simulink model "vehicle_lat_dyn_sim"  (Simulink 9.1)
settings: Solver=ode45  StartTime=0.0  StopTime=Tend  RelTol=1e-3
values from neighbouring files (symbols this model uses):
  alfaf0 = 0    [dati2.m]    (also in vehicle_lat_dyn_main.m)
  alfar0 = 0    [dati2.m]    (also in vehicle_lat_dyn_main.m)
  bf = 12    [data_vehicle.m]    (also in dati.m; dati2.m)
  br = 14    [data_vehicle.m]    (also in dati.m = 18; dati2.m = 18)
  Cd = .3    (= 0.3)    [data_vehicle.m]    (also in dati.m; dati2.m)
  Cf = 1.3    [data_vehicle.m]    (also in dati.m; dati2.m)
  Cr = 1.3    [data_vehicle.m]    (also in dati.m; dati2.m)
  df = 0.95    [data_vehicle.m]    (also in dati.m; dati2.m)
  dr = 1    [data_vehicle.m]    (also in dati.m = 1.1; dati2.m = 1.1)
  dt_save = 1e-2    (= 0.01)    [dati2.m]    (also in vehicle_lat_dyn_main.m)
  Ef = -0.1    [data_vehicle.m]    (also in dati.m; dati2.m)
  Er = -0.1    [data_vehicle.m]    (also in dati.m; dati2.m)
  fv = .02    (= 0.02)    [data_vehicle.m]    (also in dati.m; dati2.m)
  Fzf = m*g*lr/l    [data_vehicle.m]    (also in dati.m = 9879.29185185; dati2.m = 9879.29185185)
  Fzr = m*g*lf/l    [data_vehicle.m]    (also in dati.m = 5811.34814815; dati2.m = 5811.34814815)
  g = 9.80665    [dati.m]    (also in dati2.m; vehicle_lat_dyn_main.m)
  gB = 2/3    (= 0.666666666667)    [data_vehicle.m]    (also in dati.m; dati2.m)
  gT = 0    [data_vehicle.m]    (also in dati.m = 1; dati2.m = 1)
  Jz = 2200    [data_vehicle.m]    (also in dati.m; dati2.m)
  L = 2    [data_vehicle.m]    (also in dati.m; dati2.m)
  lf = 1    [data_vehicle.m]    (also in dati.m; dati2.m)
  lr = l-lf    (= 1.7)    [data_vehicle.m]    (also in dati.m; dati2.m)
  m = 1600    [data_vehicle.m]    (also in dati.m; dati2.m)
  mu = 1    [data_vehicle.m]    (also in dati.m; dati2.m)
  psi0 = 0    [dati2.m]    (also in vehicle_lat_dyn_main.m)
  psip0 = 0    [dati2.m]    (also in vehicle_lat_dyn_main.m)
  rho = 1.2    [data_vehicle.m]    (also in dati.m; dati2.m)
  S = 2    [data_vehicle.m]    (also in dati.m; dati2.m)
  vy0 = 0    [dati2.m]    (also in vehicle_lat_dyn_main.m)
  XG0 = 0    [dati2.m]    (also in vehicle_lat_dyn_main.m)
  YG0 = 0    [dati2.m]    (also in vehicle_lat_dyn_main.m)
undefined symbols (not defined in the file or in its folder): axh, deltah, vxh
settings Model: Creator=mic  LastModifiedBy=jdrjk
settings DataIOCC: SaveFormat=StructureWithTime  SaveOutput=off  SignalLogging=off  DSMLogging=off  OutputOption=SpecifiedOutputTimes  OutputTimes=[0:dt_save:Tend]
settings DebuggingCC: UnderspecifiedInitializationDetection=Simplified  MergeDetectMultiDrivingBlocksExec=error  SFUnexpectedBacktrackingDiag=error  SFNoUnconditionalDefaultTransitionDiag=error
settings HardwareCC: ProdBitPerPointer=64  ProdLargestAtomicFloat=Float  ProdIntDivRoundTo=Zero  ProdEndianess=LittleEndian  ProdHWDeviceType=Specified
settings ModelReferenceCC: PropagateSignalLabelsOutOfModel=on
settings GRTTargetCC: TargetLangStandard=C99 (ISO)  CombineOutputUpdateFcns=on  GRTInterface=off
settings ConfigComp: CovMetricSettings=dwe  CovHtmlReporting=off  CovSaveCumulativeToWorkspaceVar=off  CovSaveSingleToWorkspaceVar=off  CovExternalEMLEnable=on

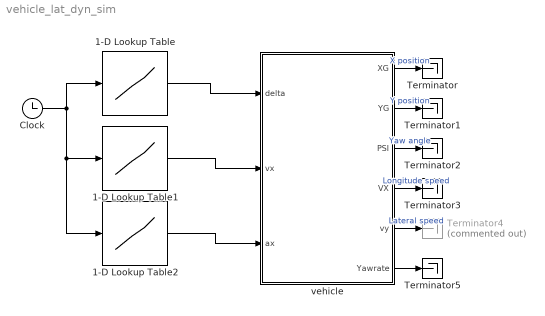
== system vehicle_lat_dyn_sim ==
  1-D Lookup Table : Lookup_n-D  NumberOfTableDimensions=1  BreakpointsForDimension1=deltah(:,1)  Table=deltah(:,2)  RndMeth=Simplest  InputSameDT=on
  1-D Lookup Table1 : Lookup_n-D  NumberOfTableDimensions=1  BreakpointsForDimension1=vxh(:,1)  Table=vxh(:,2)  RndMeth=Simplest  InputSameDT=on
  1-D Lookup Table2 : Lookup_n-D  NumberOfTableDimensions=1  BreakpointsForDimension1=axh(:,1)  Table=axh(:,2)  RndMeth=Simplest  InputSameDT=on
  Clock : Clock
  Terminator{,1..3,5} (5 alike) : Terminator
  Terminator4 : Terminator  Commented=on
  vehicle : Subsystem
  wires:
  Clock/1 -> 1-D Lookup Table2/1, 1-D Lookup Table1/1, 1-D Lookup Table/1
  1-D Lookup Table1/1 -> vehicle/2(vx)
  1-D Lookup Table2/1 -> vehicle/3(ax)
  1-D Lookup Table/1 -> vehicle/1(delta)
  vehicle/1(XG) -> Terminator/1  "X position"
  vehicle/2(YG) -> Terminator1/1  "Y position"
  vehicle/3(PSI) -> Terminator2/1  "Yaw angle"
  vehicle/4(VX) -> Terminator3/1  "Longitude speed"
  vehicle/5(vy) -> Terminator4/1  "Lateral speed"
  vehicle/6("Yawrate ") -> Terminator5/1

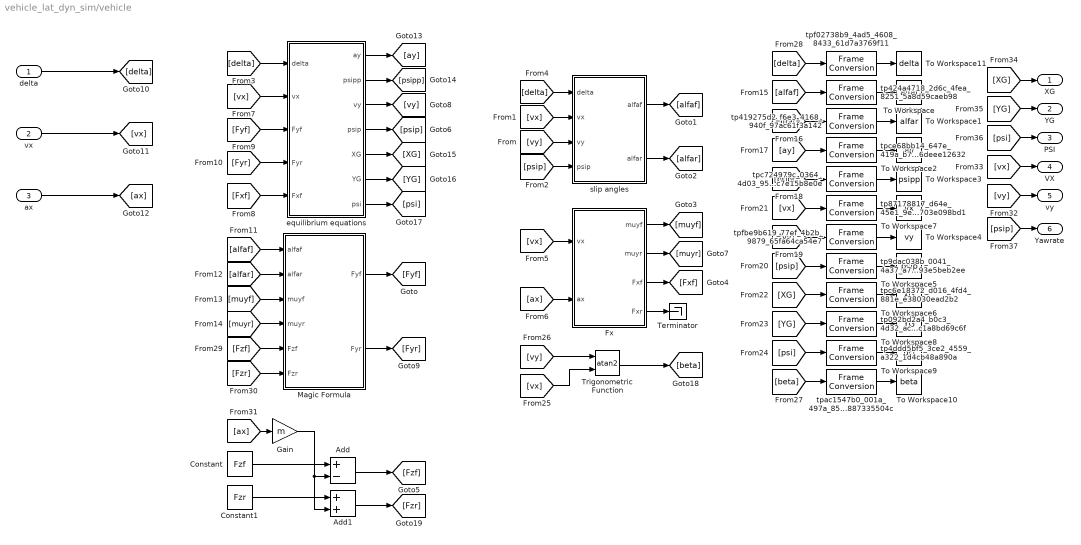
== system vehicle_lat_dyn_sim/vehicle ==
  delta : Inport
  vx : Inport  Port=2
  ax : Inport  Port=3
  Add : Sum  Inputs=+-
  Add1 : Sum
  Constant : Constant  Value=Fzf
  Constant1 : Constant  Value=Fzr
  Fx : Subsystem
  Gain : Gain  Gain=m
  Magic Formula : Subsystem
  Terminator : Terminator
  To Workspace : ToWorkspace  VariableName=alfaf  SampleTime=dt_save
  To Workspace1 : ToWorkspace  VariableName=alfar  SampleTime=dt_save
  To Workspace10 : ToWorkspace  VariableName=beta  SampleTime=dt_save
  To Workspace11 : ToWorkspace  VariableName=delta  SampleTime=dt_save
  To Workspace2 : ToWorkspace  VariableName=ay  SampleTime=dt_save
  To Workspace3 : ToWorkspace  VariableName=psipp  SampleTime=dt_save
  To Workspace4 : ToWorkspace  VariableName=vy  SampleTime=dt_save
  To Workspace5 : ToWorkspace  VariableName=psip  SampleTime=dt_save
  To Workspace6 : ToWorkspace  VariableName=XG  SampleTime=dt_save
  To Workspace7 : ToWorkspace  VariableName=vx  SampleTime=dt_save
  To Workspace8 : ToWorkspace  VariableName=YG  SampleTime=dt_save
  To Workspace9 : ToWorkspace  VariableName=psi  SampleTime=dt_save
  Trigonometric Function : Trigonometry  Operator=atan2
  equilibrium equations : Subsystem
  slip angles : Subsystem
  tp092bd2a4_b0c3_4d32_ac59_7c1a8bd69c6f : FrameConversion  OutFrame=Sample-based
  tp419275d2_f6e3_4168_940f_97ac61f3a142 : FrameConversion  OutFrame=Sample-based
  tp424a4718_2d6c_4fea_8251_5a8d59caeb98 : FrameConversion  OutFrame=Sample-based
  tp4ddd5bf5_3ce2_4559_a322_1d4cb48a890a : FrameConversion  OutFrame=Sample-based
  tp87178817_d64e_45e1_9e30_db703e098bd1 : FrameConversion  OutFrame=Sample-based
  tp9dac038b_0041_4a37_a752_0593e5beb2ee : FrameConversion  OutFrame=Sample-based
  tpac1547b0_001a_497a_857c_68887335504c : FrameConversion  OutFrame=Sample-based
  tpc6e18372_d016_4fd4_881e_e38030ead2b2 : FrameConversion  OutFrame=Sample-based
  tpc724979c_0364_4d03_952a_37c7e15b8e0e : FrameConversion  OutFrame=Sample-based
  tpce68bb14_647e_419a_b744_5f6deee12632 : FrameConversion  OutFrame=Sample-based
  tpf02738b9_4ad5_4608_8433_61d7a3769f11 : FrameConversion  OutFrame=Sample-based
  tpfbe9b619_77ef_4b2b_9879_65fa64ca54e7 : FrameConversion  OutFrame=Sample-based
  XG : Outport
  YG : Outport  Port=2
  PSI : Outport  Port=3
  VX : Outport  Port=4
  vy : Outport  Port=5
  "Yawrate " : Outport  Port=6
  wires:
  [vx] -> VX/1
  [psi] -> PSI/1
  [XG] -> XG/1
  [YG] -> YG/1
  [vy] -> vy/1
  [vx] -> equilibrium equations/2(vx)
  Magic Formula/2(Fyr) -> [Fyr]
  slip angles/1(alfaf) -> [alfaf]
  equilibrium equations/4(psip) -> [psip]
  [delta] -> equilibrium equations/1(delta)
  [vx] -> slip angles/2(vx)
  [ax] -> Fx/2(ax)
  Fx/4(Fxr) -> Terminator/1
  [Fxf] -> equilibrium equations/5(Fxf)
  [alfar] -> Magic Formula/2(alfar)
  [muyf] -> Magic Formula/3(muyf)
  [vy] -> slip angles/3(vy)
  [muyr] -> Magic Formula/4(muyr)
  slip angles/2(alfar) -> [alfar]
  Magic Formula/1(Fyf) -> [Fyf]
  [Fyf] -> equilibrium equations/3(Fyf)
  equilibrium equations/3(vy) -> [vy]
  [psip] -> slip angles/4(psip)
  [Fyr] -> equilibrium equations/4(Fyr)
  [vx] -> Fx/1(vx)
  delta/1 -> [delta]
  vx/1 -> [vx]
  Fx/1(muyf) -> [muyf]
  [alfaf] -> Magic Formula/1(alfaf)
  [delta] -> slip angles/1(delta)
  Fx/2(muyr) -> [muyr]
  Fx/3(Fxf) -> [Fxf]
  [delta] -> tpf02738b9_4ad5_4608_8433_61d7a3769f11/1
  tpf02738b9_4ad5_4608_8433_61d7a3769f11/1 -> To Workspace11/1
  [ay] -> tpce68bb14_647e_419a_b744_5f6deee12632/1
  equilibrium equations/7(psi) -> [psi]
  ax/1 -> [ax]
  [alfar] -> tp419275d2_f6e3_4168_940f_97ac61f3a142/1
  [alfaf] -> tp424a4718_2d6c_4fea_8251_5a8d59caeb98/1
  tpce68bb14_647e_419a_b744_5f6deee12632/1 -> To Workspace2/1
  [psipp] -> tpc724979c_0364_4d03_952a_37c7e15b8e0e/1
  equilibrium equations/2(psipp) -> [psipp]
  [vy] -> Trigonometric Function/1
  [Fzf] -> Magic Formula/5(Fzf)
  Gain/1 -> Add1/2, Add/2
  tp424a4718_2d6c_4fea_8251_5a8d59caeb98/1 -> To Workspace/1
  [beta] -> tpac1547b0_001a_497a_857c_68887335504c/1
  equilibrium equations/6(YG) -> [YG]
  Add1/1 -> [Fzr]
  tpac1547b0_001a_497a_857c_68887335504c/1 -> To Workspace10/1
  equilibrium equations/1(ay) -> [ay]
  Constant/1 -> Add/1
  equilibrium equations/5(XG) -> [XG]
  Constant1/1 -> Add1/1
  [Fzr] -> Magic Formula/6(Fzr)
  Trigonometric Function/1 -> [beta]
  Add/1 -> [Fzf]
  [vx] -> Trigonometric Function/2
  [ax] -> Gain/1
  tp419275d2_f6e3_4168_940f_97ac61f3a142/1 -> To Workspace1/1
  tp092bd2a4_b0c3_4d32_ac59_7c1a8bd69c6f/1 -> To Workspace8/1
  tp4ddd5bf5_3ce2_4559_a322_1d4cb48a890a/1 -> To Workspace9/1
  tpc724979c_0364_4d03_952a_37c7e15b8e0e/1 -> To Workspace3/1
  [psip] -> tp9dac038b_0041_4a37_a752_0593e5beb2ee/1
  tp87178817_d64e_45e1_9e30_db703e098bd1/1 -> To Workspace7/1
  tpc6e18372_d016_4fd4_881e_e38030ead2b2/1 -> To Workspace6/1
  [vy] -> tpfbe9b619_77ef_4b2b_9879_65fa64ca54e7/1
  tpfbe9b619_77ef_4b2b_9879_65fa64ca54e7/1 -> To Workspace4/1
  [XG] -> tpc6e18372_d016_4fd4_881e_e38030ead2b2/1
  [YG] -> tp092bd2a4_b0c3_4d32_ac59_7c1a8bd69c6f/1
  [vx] -> tp87178817_d64e_45e1_9e30_db703e098bd1/1
  tp9dac038b_0041_4a37_a752_0593e5beb2ee/1 -> To Workspace5/1
  [psi] -> tp4ddd5bf5_3ce2_4559_a322_1d4cb48a890a/1
  [psip] -> "Yawrate "/1

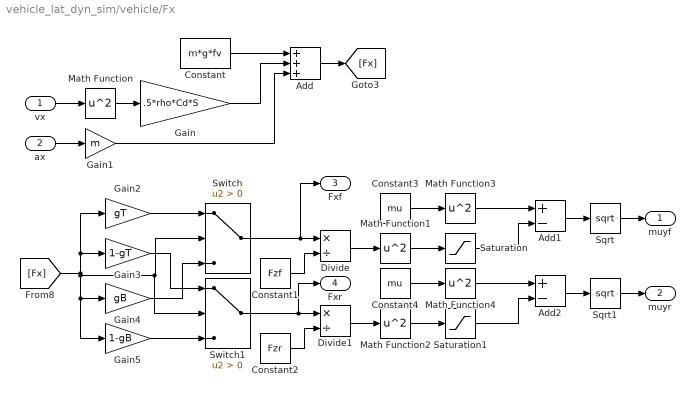
== system vehicle_lat_dyn_sim/vehicle/Fx ==
  vx : Inport
  ax : Inport  Port=2
  Add : Sum  Inputs=+++
  Add1 : Sum  Inputs=+-
  Add2 : Sum  Inputs=+-
  Constant : Constant  Value=m*g*fv
  Constant1 : Constant  Value=Fzf
  Constant2 : Constant  Value=Fzr
  Constant3 : Constant  Value=mu
  Constant4 : Constant  Value=mu
  Divide : Product  Inputs=*/
  Divide1 : Product  Inputs=*/
  Gain : Gain  Gain=.5*rho*Cd*S
  Gain1 : Gain  Gain=m
  Gain2 : Gain  Gain=gT
  Gain3 : Gain  Gain=1-gT
  Gain4 : Gain  Gain=gB
  Gain5 : Gain  Gain=1-gB
  Math Function{,1..4} (5 alike) : Math  Operator=square  SaturateOnIntegerOverflow=on
  Saturation : Saturate  UpperLimit=1  LowerLimit=0
  Saturation1 : Saturate  UpperLimit=1  LowerLimit=0
  Sqrt : Sqrt  SaturateOnIntegerOverflow=on
  Sqrt1 : Sqrt  SaturateOnIntegerOverflow=on
  Switch : Switch  Criteria=u2 > Threshold
  Switch1 : Switch  Criteria=u2 > Threshold
  muyf : Outport
  muyr : Outport  Port=2
  Fxf : Outport  Port=3
  Fxr : Outport  Port=4
  wires:
  Constant/1 -> Add/1
  Gain4/1 -> Switch/3
  Add/1 -> [Fx]
  [Fx] -> Gain2/1, Gain3/1, Switch1/2, Switch/2, Gain5/1, Gain4/1
  Gain3/1 -> Switch1/1
  Gain5/1 -> Switch1/3
  Gain1/1 -> Add/3
  Math Function/1 -> Gain/1
  Gain2/1 -> Switch/1
  Gain/1 -> Add/2
  ax/1 -> Gain1/1
  vx/1 -> Math Function/1
  Switch/1 -> Fxf/1, Divide/1
  Switch1/1 -> Fxr/1, Divide1/1
  Constant1/1 -> Divide/2
  Constant2/1 -> Divide1/2
  Constant3/1 -> Math Function3/1
  Divide/1 -> Math Function1/1
  Divide1/1 -> Math Function2/1
  Math Function1/1 -> Saturation/1
  Math Function2/1 -> Saturation1/1
  Constant4/1 -> Math Function4/1
  Saturation1/1 -> Add2/2
  Saturation/1 -> Add1/2
  Add1/1 -> Sqrt/1
  Add2/1 -> Sqrt1/1
  Sqrt1/1 -> muyr/1
  Sqrt/1 -> muyf/1
  Math Function3/1 -> Add1/1
  Math Function4/1 -> Add2/1

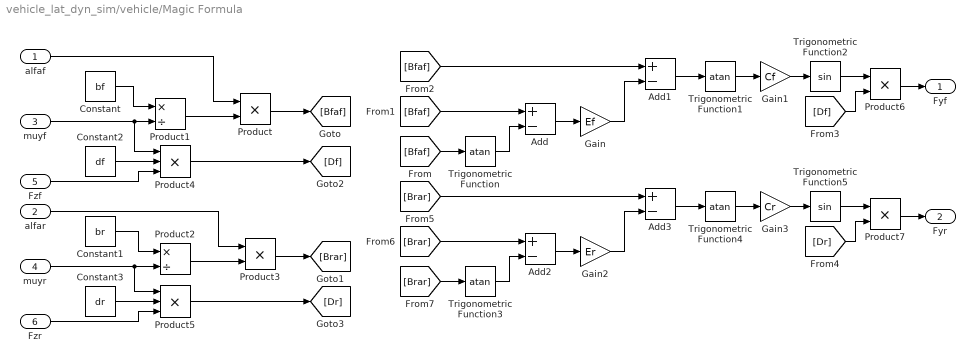
== system vehicle_lat_dyn_sim/vehicle/Magic Formula ==
  alfaf : Inport
  alfar : Inport  Port=2
  muyf : Inport  Port=3
  muyr : Inport  Port=4
  Fzf : Inport  Port=5
  Fzr : Inport  Port=6
  Add{,1..3} (4 alike) : Sum  Inputs=+-
  Constant : Constant  Value=bf
  Constant1 : Constant  Value=br
  Constant2 : Constant  Value=df
  Constant3 : Constant  Value=dr
  Gain : Gain  Gain=Ef
  Gain1 : Gain  Gain=Cf
  Gain2 : Gain  Gain=Er
  Gain3 : Gain  Gain=Cr
  Product{,3,6..7} (4 alike) : Product
  Product1 : Product  Inputs=*/
  Product2 : Product  Inputs=*/
  Product4 : Product  Inputs=3
  Product5 : Product  Inputs=3
  Trigonometric Function{,1,3..4} (4 alike) : Trigonometry  Operator=atan
  Trigonometric Function2 : Trigonometry
  Trigonometric Function5 : Trigonometry
  Fyf : Outport
  Fyr : Outport  Port=2
  wires:
  Constant/1 -> Product1/1
  muyf/1 -> Product4/1, Product1/2
  Constant1/1 -> Product2/1
  muyr/1 -> Product5/1, Product2/2
  Product1/1 -> Product/2
  alfaf/1 -> Product/1
  Product2/1 -> Product3/2
  alfar/1 -> Product3/1
  Product/1 -> [Bfaf]
  Product3/1 -> [Brar]
  Constant2/1 -> Product4/2
  Constant3/1 -> Product5/2
  Product4/1 -> [Df]
  Product5/1 -> [Dr]
  [Bfaf] -> Trigonometric Function/1
  Trigonometric Function/1 -> Add/2
  [Bfaf] -> Add/1
  Add/1 -> Gain/1
  Gain/1 -> Add1/2
  [Bfaf] -> Add1/1
  Add1/1 -> Trigonometric Function1/1
  Trigonometric Function1/1 -> Gain1/1
  Gain1/1 -> Trigonometric Function2/1
  Trigonometric Function2/1 -> Product6/1
  [Df] -> Product6/2
  Product6/1 -> Fyf/1
  [Dr] -> Product7/2
  Trigonometric Function5/1 -> Product7/1
  Gain3/1 -> Trigonometric Function5/1
  Trigonometric Function4/1 -> Gain3/1
  Add3/1 -> Trigonometric Function4/1
  [Brar] -> Add3/1
  Gain2/1 -> Add3/2
  Add2/1 -> Gain2/1
  [Brar] -> Add2/1
  Trigonometric Function3/1 -> Add2/2
  [Brar] -> Trigonometric Function3/1
  Product7/1 -> Fyr/1
  Fzf/1 -> Product4/3
  Fzr/1 -> Product5/3

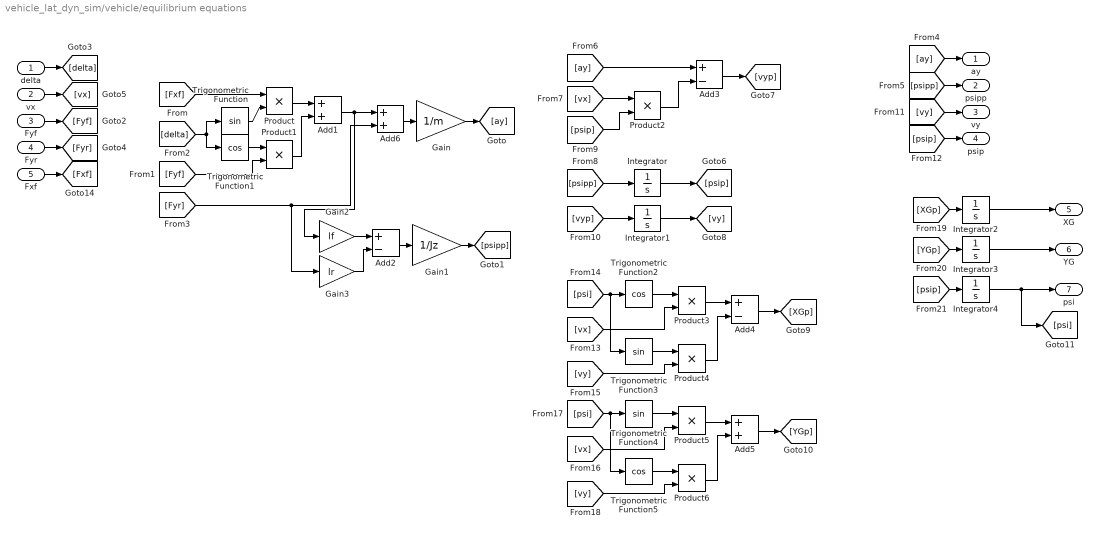
== system vehicle_lat_dyn_sim/vehicle/equilibrium equations ==
  delta : Inport
  vx : Inport  Port=2
  Fyf : Inport  Port=3
  Fyr : Inport  Port=4
  Fxf : Inport  Port=5
  Add1 : Sum
  Add2 : Sum  Inputs=+-
  Add3 : Sum  Inputs=+-
  Add4 : Sum  Inputs=+-
  Add5 : Sum
  Add6 : Sum
  Gain : Gain  Gain=1/m
  Gain1 : Gain  Gain=1/Jz
  Gain2 : Gain  Gain=lf
  Gain3 : Gain  Gain=lr
  Integrator : Integrator  InitialCondition=psip0  ContinuousStateAttributes='yaw_rate'
  Integrator1 : Integrator  InitialCondition=vy0  ContinuousStateAttributes='speed_y'
  Integrator2 : Integrator  InitialCondition=XG0  ContinuousStateAttributes='XG'
  Integrator3 : Integrator  InitialCondition=YG0  ContinuousStateAttributes='YG'
  Integrator4 : Integrator  InitialCondition=psi0  ContinuousStateAttributes='yaw'
  Product{,1..6} (7 alike) : Product
  Trigonometric Function : Trigonometry
  Trigonometric Function1 : Trigonometry  Operator=cos
  Trigonometric Function2 : Trigonometry  Operator=cos
  Trigonometric Function3 : Trigonometry
  Trigonometric Function4 : Trigonometry
  Trigonometric Function5 : Trigonometry  Operator=cos
  ay : Outport
  psipp : Outport  Port=2
  vy : Outport  Port=3
  psip : Outport  Port=4
  XG : Outport  Port=5
  YG : Outport  Port=6
  psi : Outport  Port=7
  wires:
  Product1/1 -> Add1/2
  Trigonometric Function/1 -> Product/2
  Add6/1 -> Gain/1
  Gain1/1 -> [psipp]
  [Fyr] -> Add6/2, Gain3/1
  Product/1 -> Add1/1
  Gain/1 -> [ay]
  [delta] -> Trigonometric Function/1, Trigonometric Function1/1
  Trigonometric Function1/1 -> Product1/1
  delta/1 -> [delta]
  [ay] -> ay/1
  [Fxf] -> Product/1
  Add1/1 -> Gain2/1, Add6/1
  Fyf/1 -> [Fyf]
  Add2/1 -> Gain1/1
  [Fyf] -> Product1/2
  Gain3/1 -> Add2/2
  Gain2/1 -> Add2/1
  Fyr/1 -> [Fyr]
  [psipp] -> psipp/1
  vx/1 -> [vx]
  [psipp] -> Integrator/1
  Integrator/1 -> [psip]
  [vx] -> Product2/1
  [psip] -> Product2/2
  [ay] -> Add3/1
  Product2/1 -> Add3/2
  Add3/1 -> [vyp]
  [vyp] -> Integrator1/1
  Integrator1/1 -> [vy]
  [vy] -> vy/1
  [psip] -> psip/1
  [psi] -> Trigonometric Function3/1, Trigonometric Function2/1
  Trigonometric Function2/1 -> Product3/1
  [vx] -> Product3/2
  Product3/1 -> Add4/1
  Trigonometric Function3/1 -> Product4/1
  [vy] -> Product4/2
  Product4/1 -> Add4/2
  Add4/1 -> [XGp]
  Add5/1 -> [YGp]
  Product6/1 -> Add5/2
  [vy] -> Product6/2
  Trigonometric Function5/1 -> Product6/1
  Product5/1 -> Add5/1
  [vx] -> Product5/2
  Trigonometric Function4/1 -> Product5/1
  [psi] -> Trigonometric Function4/1, Trigonometric Function5/1
  [XGp] -> Integrator2/1
  Integrator2/1 -> XG/1
  Integrator3/1 -> YG/1
  [YGp] -> Integrator3/1
  Integrator4/1 -> [psi], psi/1
  [psip] -> Integrator4/1
  Fxf/1 -> [Fxf]

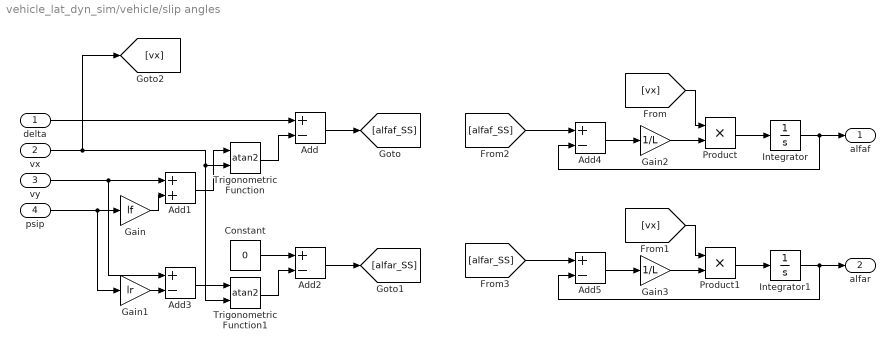
== system vehicle_lat_dyn_sim/vehicle/slip angles ==
  delta : Inport
  vx : Inport  Port=2
  vy : Inport  Port=3
  psip : Inport  Port=4
  Add{,2..5} (5 alike) : Sum  Inputs=+-
  Add1 : Sum
  Constant : Constant  Value=0
  Gain : Gain  Gain=lf
  Gain1 : Gain  Gain=lr
  Gain2 : Gain  Gain=1/L
  Gain3 : Gain  Gain=1/L
  Integrator : Integrator  InitialCondition=alfaf0  ContinuousStateAttributes='slip_angle_f'
  Integrator1 : Integrator  InitialCondition=alfar0  ContinuousStateAttributes='slip_angle_r'
  Product : Product
  Product1 : Product
  Trigonometric Function : Trigonometry  Operator=atan2
  Trigonometric Function1 : Trigonometry  Operator=atan2
  alfaf : Outport
  alfar : Outport  Port=2
  wires:
  vy/1 -> Add3/1, Add1/1
  Constant/1 -> Add2/1
  Add3/1 -> Trigonometric Function1/1
  Trigonometric Function/1 -> Add/2
  Gain1/1 -> Add3/2
  vx/1 -> [vx], Trigonometric Function1/2, Trigonometric Function/2
  psip/1 -> Gain1/1, Gain/1
  Add1/1 -> Trigonometric Function/1
  Gain/1 -> Add1/2
  Trigonometric Function1/1 -> Add2/2
  delta/1 -> Add/1
  Add/1 -> [alfaf_SS]
  Add2/1 -> [alfar_SS]
  [alfaf_SS] -> Add4/1
  [alfar_SS] -> Add5/1
  Add4/1 -> Gain2/1
  Add5/1 -> Gain3/1
  Gain2/1 -> Product/2
  Gain3/1 -> Product1/2
  [vx] -> Product/1
  [vx] -> Product1/1
  Product/1 -> Integrator/1
  Integrator/1 -> Add4/2, alfaf/1
  Product1/1 -> Integrator1/1
  Integrator1/1 -> alfar/1, Add5/2
